simulink model "Phase1_Mark2"  (R2024b)
settings: Solver=ode23tb  StartTime=0.0  StopTime=inf  FixedStep=.001  RelTol=1e-1
model workspace (MAT data in the model file):
  A_mu = 10
  B_reff = 8.386
  CONVERTER_DATA = [0 0.1 0.2 0.3 0.4 0.5 0.6 0.7 0.8 0.81 0.82 0.83 ... (63 elements, 21x3)]
  Cps = 2
  Cz = 7766.25
  DOWN_TABLE = [0 0 0 0 0 0 5 5 7.5 7.5 15 15 ... (30 elements, 6x5)]
  DOWN_TH_BP = [0 5 40 50 90 100]
  D_reff = 0.25826
  EMAP = [-40 215 245 264 264 267 267 267 267 267 -44 117 ... (110 elements, 10x11)]
  F0z = [6086.4 4324.8]
  F_reff = 0.07394
  F_zmax = 10000
  F_zmin = 100
  F_zo = 4000
  Kz = 48000
  MF : object (value not decoded)
  NCyl = 6
  NE_VEC = [800 1200 1600 2000 2400 2800 3200 3600 4000 4400 4800]
  Pstd = 101325
  Rair = 287
  SUS : object (value not decoded)
  TH_VEC = [0; 20; 30; 40; 50; 60; 70; 80; 90; 100]
  TWAITdn = 1.25
  TWAITup = 0.1
  Tin = [1 2 3 4 5 6 7 8 9 10 2 2 ... (20 elements, 10x2)]
  Tstd = 293.15
  UP_TABLE = [7.5 7.5 15 25 40 40 25 25 35 45 70 80 ... (30 elements, 6x5)]
  UP_TH_BP = [0 25 35 50 90 100]
  VEH : object (value not decoded)
  V_o = 16.7
  V_xlow = 1
  Vd = 0.00346
  WH : object (value not decoded)
  a = 1.515
  alpha_max = 1.5
  alpha_min = -1.5
  b = 1.504
  c_zo = 209651
  epsilon = 0.1
  f_air = [0 0 0 0 0 0 0 0 0 0 0 0 ... (256 elements, 16x16)]
  f_co = [0 0 0 0 0 0 0 0 0 0 0 0 ... (256 elements, 16x16)]
  f_co2 = [0 0 0 0 0 0 0 0 0 0 0 0 ... (256 elements, 16x16)]
  f_eff = [352.135682859 352.135682859 320.724378192 303.655312657 295.930136708 291.240087194 291.240271258 291.240312459 291.240275452 291.240198499 291.240100781 291.240018769 ... (256 elements, 16x16)]
  f_fuel = [0 0 0 0 0 0 0 0 0 0 0 0 ... (256 elements, 16x16)]
  f_hc = [0 0 0 0 0 0 0 0 0 0 0 0 ... (256 elements, 16x16)]
  f_nox = [0 0 0 0 0 0 0 0 0 0 0 0 ... (256 elements, 16x16)]
  f_pm = [0 0 0 0 0 0 0 0 0 0 0 0 ... (256 elements, 16x16)]
  f_susp_axl_bp = [1 2]
  f_susp_dz_bp = [-4 -0.14 -0.13 -0.12 -0.11 -0.1 -0.09 -0.08 -0.07 -0.06 -0.05 -0.04 ... (31 elements, 1x31)]
  f_susp_dzdot_bp = [-4 -0.14 -0.13 -0.12 -0.11 -0.1 -0.09 -0.08 -0.07 -0.06 -0.05 -0.04 ... (31 elements, 1x31)]
  f_susp_fmz = [-213379.591456 -28099.591456 -27619.591456 -27139.591456 -26659.591456 -26179.591456 -25699.591456 -25219.591456 -24739.591456 -24259.591456 -23779.591456 -23299.591456 ... (468968 elements, 31x31x61x2x4)]
  f_susp_geom = [-0.832564012244 0.043269987756 0.045538987756 0.047807987756 0.050076987756 0.052345987756 0.054614987756 0.056883987756 0.059152987756 0.061421987756 0.063690987756 0.065959987756 ... (11346 elements, 31x61x2x3)]
  f_susp_strgdelta_bp = [-0.523598775598 -0.506145483078 -0.488692190558 -0.471238898038 -0.453785605519 -0.436332312999 -0.418879020479 -0.401425727959 -0.383972435439 -0.366519142919 -0.349065850399 -0.331612557879 ... (61 elements, 1x61)]
  f_tbrake = [0 76.8593923996 105.140482948 131.533638111 157.926793274 176.658631717 176.65727296 176.656856686 176.656879077 176.657093756 176.657404516 176.65772406 ... (256 elements, 16x16)]
  f_tbrake_n_bpt = [0 649.519052838 912.419621844 1175.32019085 1438.22075986 1701.12132886 1964.02189787 2226.92246687 2489.82303588 2752.72360489 3015.62417389 3278.5247429 ... (16 elements, 1x16)]
  f_tbrake_t_bpt = [0 34.6410161514 61.0341713143 87.4273264773 113.82048164 140.213636803 166.606791966 192.999947129 219.393102292 245.786257455 272.179412618 298.572567781 ... (16 elements, 1x16)]
  f_texh = [766.752464599 766.752464599 786.17542386 801.679939032 884.591982581 910.574397722 910.571871054 910.570774534 910.570601632 910.570821151 910.571247242 910.571639815 ... (256 elements, 16x16)]
  f_twc_eff_co = [0.17 0.25 0.45 0.99 0.99 0.99 0.99]
  f_twc_eff_hc = [0.21 0.375 0.75 0.98 0.98 0.98 0.98]
  f_twc_eff_lam = [0.909090909 0.944055944 0.979020979 1 1.013986014 1.048951049 1.083916084]
  f_twc_eff_nox = [0.98 0.98 0.98 0.97 0.05 0.02 0]
  h = 0.134
  k_z = 50
  kappa_max = 1.5
  kappa_min = -1.5
  lam_Cx = 1
  lam_Cy = 1
  lam_Cz = 1
  lam_Ex = 1
  lam_Ey = 1
  lam_F_zo = 1
  lam_Hx = 1
  lam_Hy = 1
  lam_Kxkappa = 1
  lam_Kyalpha = 1
  lam_Kygamma = 1
  lam_Kzgamma = 1
  lam_Mr = 1
  lam_Mx = 1
  lam_My = 1
  lam_S = 1
  lam_VMx = 1
  lam_Vx = 1
  lam_Vy = 1
  lam_Vykappa = 1
  lam_muV = 0
  lam_mux = 1
  lam_muy = 1
  lam_t = 1
  lam_xalpha = 1
  lam_ykappa = 1
  numWheel = 4
  p_Cx1 = 1.579
  p_Cy1 = 1.3332
  p_Dx1 = 1.0422
  p_Dx2 = -0.08285
  p_Dx3 = 0
  p_Dy1 = 0.8784
  p_Dy2 = -0.06445
  p_Dy3 = 0
  p_Ex1 = 0.11185
  p_Ex2 = 0.3127
  p_Ex3 = 0
  p_Ex4 = 0.001603
  p_Ey1 = -0.8227
  p_Ey2 = -0.6062
  p_Ey3 = 0.09825
  p_Ey4 = -6.546
  p_Ey5 = 0
  p_Fz1 = 0.7098
  p_Hx1 = 0.00021585
  p_Hx2 = 0.0011538
  p_Hy1 = -0.0018043
  p_Hy2 = 0.003518
  p_Kx1 = 21.69
  p_Kx2 = 13.774
  p_Kx3 = -0.4119
  p_Ky1 = -15.314
  p_Ky2 = 1.7044
  p_Ky3 = 0.36986
  p_Ky4 = 1.9896
  p_Ky5 = 0
  p_Ky6 = -0.9004
  p_Ky7 = -0.2328
  p_Vx1 = 1.5973e-05
  p_Vx2 = 0.0001043
  p_Vy1 = -0.006642
  p_Vy2 = 0.03597
  p_Vy3 = -0.1621
  p_Vy4 = -0.4908
  p_pmx1 = 0
  p_px1 = -0.3489
  p_px2 = 0.382
  p_px3 = -0.09634
  p_px4 = 0.06447
  p_py1 = -0.6249
  p_py2 = -0.06535
  p_py3 = -0.1668
  p_py4 = 0.2834
  p_py5 = 0
  path : object (value not decoded)
  pio = 220000
  q_Fcx = 0
  q_Fz2 = 15.4
  q_Fzy = 0
  q_reo = 0.9974
  q_sx1 = -0.007764
  q_sx10 = 0.2824
  q_sx11 = 5.349
  q_sx12 = 0
  q_sx13 = 0
  q_sx14 = 0
  q_sx2 = 1.1915
  q_sx3 = 0.013948
  q_sx4 = 4.912
  q_sx5 = 1.02
  q_sx6 = 22.83
  q_sx7 = 0.7104
  q_sx8 = -0.023393
  q_sx9 = 0.6581
  q_sy1 = 0.00702
  q_sy2 = 0
  q_sy3 = 0.001515
  q_sy4 = 8.514e-05
  q_sy5 = 0
  q_sy6 = 0
  q_sy7 = 0.9008
  q_sy8 = -0.4089
  q_v1 = 0.0007742
  q_v2 = 0.04667
  r_Bx1 = 12.531
  r_Bx2 = 9.532
  r_Bx3 = 0
  r_By1 = 10.615
  r_By2 = 7.705
  r_By3 = 3.433e-06
  r_By4 = 0
  r_Cx1 = 1.019
  r_Cy1 = 1.0585
  r_Ex1 = -0.4487
  r_Ex2 = -0.4726
  r_Ey1 = 0.3132
  r_Ey2 = 7.63e-06
  r_Hx1 = 0.0002374
  r_Hy1 = 0.011646
  r_Hy2 = 7.63e-06
  r_Vy1 = 0.05654
  r_Vy2 = 7.63e-06
  r_Vy3 = 0
  r_Vy4 = 99.9
  r_Vy5 = 2
  r_Vy6 = 15.814
  r_o = 0.3135
  reqTmaxT = [nan 0.285774810084 0.647179872268 nan nan nan nan nan nan nan nan nan ... (168 elements, 21x8)]
  vehSpd = [0 2.77777777778 5.55555555556 8.33333333333 11.1111111111 13.8888888889 16.6666666667 19.4444444444 22.2222222222 25 27.7777777778 30.5555555556 ... (21 elements, 1x21)]
  vehWidth = 2
  w = 1
symbols that are objects in the model workspace (value not decoded): VEH
undefined symbols (not defined in the file or in its folder): Fzz, Fzzdot, InertFrm, pFz, psi, vdyntiremask, x_o, zdotFz, zFz
(part 4 of 24)

== system Phase1_Mark2/Longitudinal Wheels 4DOF/Tires/Fiala ==
  AxlTrq : Inport
  BrkPrs : Inport  Port=2
  Vx : Inport  Port=3
  Vy : Inport  Port=4
  r : Inport  Port=5
  Camber : Inport  Port=6
  TirePrs : Inport  Port=7
  Fz : Inport  Port=8
  Friction : Inport  Port=9
  Ground : Inport  Port=10
  Fiala Tire : Subsystem  InitFcn=%vdyntiremask(gcb,'updateExtAPIButtons');  mask(Fiala Wheel 2DOF){UNLOADED_RADIUS=0.309384029954441, omegao=0, IYY=0.740633832792491, br=1e-3, tireType=User defined, BrakeType=Disc, rollingType=Pressure and velocity, vertType=None, Ckappa=1e4, Calpha=7e4, Cgamma=1e3, muMin=.8, muMax=.9, Lrelx=.01, Lrely=.01, NOMPRES=220000, LONGVL=16, aMy=8e-4, bMy=.001, cMy=1.6e-4, alphaMy=-0.003, betaMy=0.97, QSY1=0.007, QSY2=0, QSY3=0.0015, QSY4=8.5e-05, QSY5=0, QSY6=0, QSY7=0.9, QSY8=-0.4, FNOMIN=4000, lam_My=1, VxMy=-20:1:20, FzMy=0:200:1e4, MyMap=[0,1114.7,4367.1,9707.2,17109,26554,38030,51524,67028,84533,1.0403e+05,1.2552e+05,1.4899e+05,1.7444e+05,2.0185e+05,2.3124e+05,2.6259e+05,2.959e+05,3.3117e+05,3.6839e+05,4.0756e+05,4.4868e+05,4.9174e+05,5.3675e+05,5.8369e+05,6.3257e+05,6.8338e+05,7.3613e+05,7.908e+05,8.474e+05,9.0593e+05,9.6638e+05,1.0288e+06,1.093e+06,1.1593e+06,1.2274e+06,1.2974e+06,1.3694e+06,1.4432e+06,1.519e+06,1.5967e+06,1.6763e+06,1.7578e+06,1.8412e+06,1.9265e+06,2.0137e+06,2.1028e+06,2.1938e+06,2.2867e+06,2.3815e+06,2.4782e+06 0,1024.5,4013.8,8921.9,15725,24406,34953,47356,61605,77694,95616,1.1537e+05,1.3694e+05,1.6032e+05,1.8553e+05,2.1254e+05,2.4135e+05,2.7197e+05,3.0438e+05,3.3859e+05,3.7459e+05,4.1238e+05,4.5196e+05,4.9333e+05,5.3647e+05,5.814e+05,6.281e+05,6.7658e+05,7.2683e+05,7.7885e+05,8.3264e+05,8.8821e+05,9.4553e+05,1.0046e+06,1.0655e+06,1.1281e+06,1.1925e+06,1.2586e+06,1.3265e+06,1.3961e+06,1.4675e+06,1.5407e+06,1.6156e+06,1.6922e+06,1.7706e+06,1.8508e+06,1.9327e+06,2.0163e+06,2.1017e+06,2.1889e+06,2.2777e+06 0,938.57,3677,8173.3,14405,22358,32020,43382,56436,71175,87593,1.0568e+05,1.2545e+05,1.4687e+05,1.6996e+05,1.947e+05,2.211e+05,2.4915e+05,2.7884e+05,3.1018e+05,3.4316e+05,3.7778e+05,4.1404e+05,4.5193e+05,4.9146e+05,5.3261e+05,5.754e+05,6.1981e+05,6.6584e+05,7.135e+05,7.6278e+05,8.1368e+05,8.6619e+05,9.2032e+05,9.7607e+05,1.0334e+06,1.0924e+06,1.153e+06,1.2152e+06,1.279e+06,1.3444e+06,1.4114e+06,1.48e+06,1.5502e+06,1.6221e+06,1.6955e+06,1.7705e+06,1.8471e+06,1.9254e+06,2.0052e+06,2.0866e+06 0,856.81,3356.7,7461.3,13151,20411,29231,39603,51520,64974,79962,96478,1.1452e+05,1.3408e+05,1.5515e+05,1.7774e+05,2.0184e+05,2.2744e+05,2.5455e+05,2.8316e+05,3.1327e+05,3.4487e+05,3.7797e+05,4.1256e+05,4.4864e+05,4.8621e+05,5.2527e+05,5.6581e+05,6.0784e+05,6.5134e+05,6.9633e+05,7.4279e+05,7.9073e+05,8.4015e+05,8.9104e+05,9.4341e+05,9.9724e+05,1.0525e+06,1.1093e+06,1.1676e+06,1.2273e+06,1.2885e+06,1.3511e+06,1.4152e+06,1.4808e+06,1.5478e+06,1.6163e+06,1.6862e+06,1.7576e+06,1.8305e+06,1.9048e+06 0,779.25,3052.9,6785.9,11960,18563,26585,36018,46856,59093,72724,87745,1.0415e+05,1.2194e+05,1.4111e+05,1.6165e+05,1.8357e+05,2.0685e+05,2.3151e+05,2.5753e+05,2.8491e+05,3.1365e+05,3.4376e+05,3.7522e+05,4.0803e+05,4.422e+05,4.7772e+05,5.1459e+05,5.5282e+05,5.9238e+05,6.333e+05,6.7556e+05,7.1916e+05,7.641e+05,8.1039e+05,8.5801e+05,9.0697e+05,9.5727e+05,1.0089e+06,1.0619e+06,1.1162e+06,1.1718e+06,1.2288e+06,1.2871e+06,1.3467e+06,1.4077e+06,1.47e+06,1.5336e+06,1.5985e+06,1.6648e+06,1.7324e+06 0,705.9,2765.5,6147.1,10834,16816,24083,32628,42446,53531,65879,79486,94348,1.1046e+05,1.2783e+05,1.4643e+05,1.6629e+05,1.8738e+05,2.0972e+05,2.3329e+05,2.5809e+05,2.8413e+05,3.114e+05,3.399e+05,3.6962e+05,4.0058e+05,4.3276e+05,4.6616e+05,5.0078e+05,5.3662e+05,5.7369e+05,6.1197e+05,6.5146e+05,6.9218e+05,7.3411e+05,7.7725e+05,8.216e+05,8.6717e+05,9.1394e+05,9.6193e+05,1.0111e+06,1.0615e+06,1.1131e+06,1.1659e+06,1.22e+06,1.2752e+06,1.3316e+06,1.3892e+06,1.4481e+06,1.5081e+06,1.5693e+06 0,636.76,2494.6,5545,9773.1,15169,21724,29432,38288,48287,59426,71700,85106,99642,1.153e+05,1.3209e+05,1.5e+05,1.6903e+05,1.8917e+05,2.1044e+05,2.3281e+05,2.563e+05,2.809e+05,3.066e+05,3.3342e+05,3.6134e+05,3.9037e+05,4.205e+05,4.5173e+05,4.8406e+05,5.1749e+05,5.5202e+05,5.8765e+05,6.2438e+05,6.622e+05,7.0111e+05,7.4112e+05,7.8223e+05,8.2442e+05,8.677e+05,9.1208e+05,9.5754e+05,1.0041e+06,1.0517e+06,1.1005e+06,1.1503e+06,1.2012e+06,1.2532e+06,1.3062e+06,1.3604e+06,1.4156e+06 0,571.82,2240.2,4979.5,8776.4,13622,19508,26430,34383,43363,53365,64388,76427,89480,1.0355e+05,1.1862e+05,1.347e+05,1.5179e+05,1.6988e+05,1.8897e+05,2.0907e+05,2.3016e+05,2.5225e+05,2.7534e+05,2.9942e+05,3.2449e+05,3.5056e+05,3.7761e+05,4.0566e+05,4.3469e+05,4.6472e+05,4.9573e+05,5.2772e+05,5.607e+05,5.9467e+05,6.2961e+05,6.6554e+05,7.0245e+05,7.4034e+05,7.7921e+05,8.1906e+05,8.5989e+05,9.017e+05,9.4448e+05,9.8824e+05,1.033e+06,1.0787e+06,1.1254e+06,1.173e+06,1.2216e+06,1.2712e+06 0,511.09,2002.3,4450.7,7844.3,12175,17436 ...(+15095 chars)], Fpl=10, Cr=1e-3, Kt=.008, Tmeas=298.15, Tamb=298.15, extTamb=off, WIDTH=0.209045013245853, bMz=0, mu_static=.3, mu_kinetic=.2, disk_abore=.05, Rm=.177, num_pads=2, drum_abore=0.0508, drum_a=0.123, drum_c=0.212, drum_r=0.15, drum_theta1=0, drum_theta2=126, brake_p_bpt=[1 11.4736842105263 21.9473684210526 32.4210526315789 42.8947368421053 53.3684210526316 63.8421052631579 74.3157894736842 84.7894736842105 95.2631578947368 105.736842105263 116.210526315789 126.684210526316 137.157894736842 147.631578947368 158.105263157895 168.578947368421 179.052631578947 189.526315789474 200], brake_n_bpt=[0 52.6315789473684 105.263157894737 157.894736842105 210.526315789474 263.157894736842 315.789473684211 368.421052631579 421.052631578947 473.684210526316 526.315789473684 578.947368421053 631.578947368421 684.210526315789 736.842105263158 789.473684210526 842.105263157895 894.736842105263 947.368421052632 1000], f_brake_t=[43.4900602404453 42.5056030554862 41.5350898940194 40.5780454442085 39.6340111501808 38.7025443887544 37.7832176914519 36.8756180088306 35.9793460143796 35.0940154454303 34.2192524787115 33.3546951383474 32.4999927342521 31.6548053290159 30.8188032315107 29.991666515561 29.1730845621415 28.362755623661 27.5603864089927 26.765691687993;498.991217495636 487.695866636631 476.560505099801 465.579679307235 454.748127933653 444.060772460445 433.51270824929 423.099196101319 412.81565427025 402.657650900201 392.620896861006 382.701238955775 372.894653477208 363.197240090814 353.605216024701 344.114910546964 334.722759712992 325.425301366216 316.219170376863 307.10109410434;954.492374750826 932.886130217776 911.585920305583 890.581313170261 869.862244717126 849.419000532136 829.242198807128 809.322774193808 789.651962526121 770.221286354971 751.0225412433 732.047782773203 713.289314220164 694.739674852612 676.391628817892 658.238154578366 640.272434863842 622.48784710877 604.877954344734 587.436496520688;1409.99353200602 1378.07639379892 1346.61133551136 1315.58294703329 1284.9763615006 1254.77722860383 1224.97168936497 1195.5463522863 1166.48827078199 1137.78492180974 1109.42418562559 1081.39432659063 1053.68397496312 1026.28210961441 999.178041611083 972.361398609768 945.822110014692 919.550392851325 893.536738312604 867.771898937035;1865.49468926121 1823.26665738007 1781.63675071715 1740.58458089631 1700.09047828407 1660.13545667552 1620.7011799228 1581.76993037878 1543.32457903786 1505.34855726451 1467.82583000789 1430.74087040806 1394.07863570608 1357.82454437621 1321.96445440427 1286.48464264117 1251.37178516554 1216.61293859388 1182.19552228048 1148.10730135338;2320.9958465164 2268.45692096121 2216.66216592293 2165.58621475934 2115.20459506754 2065.49368474721 2016.43067048064 1967.99350847127 1920.16088729373 1872.91219271928 1826.22747439018 1780.08741422549 1734.47329644903 1689.36697913801 1644.75086719747 1600.60788667257 1556.92146031639 1513.67548433643 1470.85430624835 1428.44270376973;2776.49700377159 2713.64718454235 2651.68758112871 2590.58784862237 2530.31871185102 2470.8519128189 2412.16016103848 2354.21708656376 2296.9971955496 2240.47582817405 2184.62911877248 2129.43395804292 2074.86795719199 2020.9094138998 1967.53727999066 1914.73113070398 1862.47113546724 1810.73803007899 1759.51309021622 1708.77810618608;3231.99816102678 3158.8374481235 3086.71299633449 3015.58948248539 2945.43282863449 2876.21014089059 2807.88965159632 2740.44066465625 2673.83350380547 2608.03946362882 2543.03076315477 2478.78050186034 2415.26261793494 2352.4518486616 2290.32369278385 2228.85437473538 2168.02081061809 2107.80057582154 2048.17187418409 1989.11350860242;3687.49931828197 3604.02771170464 3521.73841154027 3440.59111634842 3360.54694541796 3281.56836896228 3203.61914215416 3126.66424274874 3050.66981206134 2975.60309908359 2901.43240753707 2828.12704567777 2755.6572786779 2683.9942834234 2613.11010557704 2542.97761876678 2473.57048576894 2404.8631215641 2336.83065815196 2269.44891101877;4143.00047553716 4049.21797528579 3956.76382674606 3865.59275021144 3775.66106220143 3686.92659703397 3599.34863271199 3512.88782084123 3427.50612031721 3343.16673453836 3259.83405191936 3177.4735894952 3096.05193942085 3015.5367181852 2935.89651837023 2857.10086279818 2779.12016091979 2701.92566730665 2625.48944211983 2549.78431343512;4598.50163279235 4494.40823886693 4391.78924195184 4290.59438407447 4190.77517898491 4092.28482510566 3995.07812326983 3899.11139893372 3804.34242857308 3710.73036999313 3618.23569630166 3526.82013331263 3436.44660016381 3347.079152947 3258.68293116342 3171.22410682959 3084.66983607064 2998.98821304921 2914.1482260877 2830.11971585147;5054.00279004754 4939.59850244808 4826.81465715762 4715.59601793749 4605.88929576838 4497.64305317735 4390.80761382767 4285.3349770262 4181.17873682896 4078.2940054479 3976.63734068395 3876.16667713006 3776.84126090677 3678.62158770879 3581.46934395661 3485.34735086099 ...(+2764 chars)], MASS=9.46491996974568, zo=0, zdoto=0, GRAVITY=-9.81, VERTICAL_DAMPING=500, VERTICAL_STIFFNESS=207885, zFz=[0 .01 .1], pFz=[10000 1000000], Fzz=[0 1e3 1e4; 0 1e4 1e5], zdotFz=[-20 0 20], Fzzdot=[500 0 -500;250 0 -250], FZMAX=10000, FZMIN=100, PRESMAX=1003118.65547859, PRESMIN=9982.11955979412, KPUMAX=1.48764378595932, KPUMIN=-1.48007456759542, ALPMAX=1.47424202250808, ALPMIN=-1.50806269049027, CAMMAX=0.173142086627737, CAMMIN=-0.173348165334087, TMIN=0, TMAX=400, aMode=2, MyRelFreqLwrLim=100*pi}
      mask prompts: UNLOADED_RADIUS "vdynblks:vehdynLatTire:blkPrm_UNLOADED_RADIUS"; omegao "vdynblks:vehdynLatTire:blkPrm_omegao"; IYY "vdynblks:vehdynLatTire:blkPrm_IYY"; br "vdynblks:vehdynLatTire:blkPrm_br"; tireType "vdynblks:vehdynLatTire:blkPrm_tireType"; BrakeType "vdynblks:vehdynLatTire:blkPrm_BrakeType"; rollingType "autoblks_shared:autoblkLongitudinalWheel:blkPrm_rollingType"; vertType "vdynblks:vehdyntireFiala:blkPrm_vertType"; Ckappa "vdynblks:vehdyntireFiala:blkPrm_Ckappa"; Calpha "vdynblks:vehdyntireFiala:blkPrm_Calpha"; Cgamma "vdynblks:vehdyntireFiala:blkPrm_Cgamma"; muMin "vdynblks:vehdyntireFiala:blkPrm_muMin"; muMax "vdynblks:vehdyntireFiala:blkPrm_muMax"; Lrelx "vdynblks:vehdyntireFiala:blkPrm_Lrelx"; Lrely "vdynblks:vehdyntireFiala:blkPrm_Lrely"; NOMPRES "autoblks_shared:autoblkLongitudinalWheel:blkPrm_NOMPRES"; LONGVL "autoblks_shared:autoblkLongitudinalWheel:blkPrm_LONGVL"; aMy "vdynblks:vehdyntireFiala:blkPrm_aMy"; bMy "vdynblks:vehdyntireFiala:blkPrm_bMy"; cMy "vdynblks:vehdyntireFiala:blkPrm_cMy"; alphaMy "vdynblks:vehdyntireFiala:blkPrm_alphaMy"; betaMy "vdynblks:vehdyntireFiala:blkPrm_betaMy"; QSY1 "autoblks_shared:autoblkLongitudinalWheel:blkPrm_QSY1"; QSY2 "autoblks_shared:autoblkLongitudinalWheel:blkPrm_QSY2"; QSY3 "autoblks_shared:autoblkLongitudinalWheel:blkPrm_QSY3"; QSY4 "autoblks_shared:autoblkLongitudinalWheel:blkPrm_QSY4"; QSY5 "autoblks_shared:autoblkLongitudinalWheel:blkPrm_QSY5"; QSY6 "autoblks_shared:autoblkLongitudinalWheel:blkPrm_QSY6"; QSY7 "autoblks_shared:autoblkLongitudinalWheel:blkPrm_QSY7"; QSY8 "autoblks_shared:autoblkLongitudinalWheel:blkPrm_QSY8"; FNOMIN "autoblks_shared:autoblkLongitudinalWheel:blkPrm_FNOMIN"; lam_My "autoblks_shared:autoblkLongitudinalWheel:blkPrm_lam_My"; VxMy "autoblks_shared:autoblkLongitudinalWheel:blkPrm_VxMy"; FzMy "autoblks_shared:autoblkLongitudinalWheel:blkPrm_FzMy"; MyMap "autoblks_shared:autoblkLongitudinalWheel:blkPrm_MyMap"; Fpl "autoblks_shared:autoblkLongitudinalWheel:blkPrm_Fpl"; Cr "autoblks_shared:autoblkLongitudinalWheel:blkPrm_Cr"; Kt "autoblks_shared:autoblkLongitudinalWheel:blkPrm_Kt"; Tmeas "autoblks_shared:autoblkLongitudinalWheel:blkPrm_Tmeas"; Tamb "autoblks_shared:autoblkLongitudinalWheel:blkPrm_Tamb"; extTamb "autoblks_shared:autoblkLongitudinalWheel:blkPrm_extTamb"; WIDTH "vdynblks:vehdynLatTire:blkPrm_WIDTH"; bMz "vdynblks:vehdyntireFiala:blkPrm_bMz"; mu_static "autoblks_shared:autoblkLongitudinalWheel:blkPrm_mu_static"; mu_kinetic "autoblks_shared:autoblkLongitudinalWheel:blkPrm_mu_kinetic"; disk_abore "autoblks_shared:autoblkLongitudinalWheel:blkPrm_disk_abore"; Rm "autoblks_shared:autoblkLongitudinalWheel:blkPrm_Rm"; num_pads "autoblks_shared:autoblkLongitudinalWheel:blkPrm_num_pads"; drum_abore "autoblks_shared:autoblkLongitudinalWheel:blkPrm_drum_abore"; drum_a "autoblks_shared:autoblkLongitudinalWheel:blkPrm_drum_a"; drum_c "autoblks_shared:autoblkLongitudinalWheel:blkPrm_drum_c"; drum_r "autoblks_shared:autoblkLongitudinalWheel:blkPrm_drum_r"; drum_theta1 "autoblks_shared:autoblkLongitudinalWheel:blkPrm_drum_theta1"; drum_theta2 "autoblks_shared:autoblkLongitudinalWheel:blkPrm_drum_theta2"; brake_p_bpt "autoblks_shared:autoblkLongitudinalWheel:blkPrm_brake_p_bpt"; brake_n_bpt "autoblks_shared:autoblkLongitudinalWheel:blkPrm_brake_n_bpt"; f_brake_t "autoblks_shared:autoblkLongitudinalWheel:blkPrm_f_brake_t"; MASS "vdynblks:vehdynLatTire:blkPrm_MASS"; zo "vdynblks:vehdynLatTire:blkPrm_zo"; zdoto "vdynblks:vehdynLatTire:blkPrm_zdoto"; GRAVITY "vdynblks:vehdynLatTire:blkPrm_GRAVITY"; VERTICAL_DAMPING "vdynblks:vehdynLatTire:blkPrm_VERTICAL_DAMPING"; VERTICAL_STIFFNESS "vdynblks:vehdynLatTire:blkPrm_VERTICAL_STIFFNESS"; zFz "vdynblks:vehdyntireFiala:blkPrm_zFz"; pFz "vdynblks:vehdyntireFiala:blkPrm_pFz"; Fzz "vdynblks:vehdyntireFiala:blkPrm_Fzz"; zdotFz "vdynblks:vehdyntireFiala:blkPrm_zdotFz"; Fzzdot "vdynblks:vehdyntireFiala:blkPrm_Fzzdot"; FZMAX "vdynblks:vehdynLatTire:blkPrm_FZMAX"; FZMIN "vdynblks:vehdynLatTire:blkPrm_FZMIN"; PRESMAX "vdynblks:vehdynLatTire:blkPrm_PRESMAX"; PRESMIN "vdynblks:vehdynLatTire:blkPrm_PRESMIN"; KPUMAX "vdynblks:vehdynLatTire:blkPrm_KPUMAX"; KPUMIN "vdynblks:vehdynLatTire:blkPrm_KPUMIN"; ALPMAX "vdynblks:vehdynLatTire:blkPrm_ALPMAX"; ALPMIN "vdynblks:vehdynLatTire:blkPrm_ALPMIN"; CAMMAX "vdynblks:vehdynLatTire:blkPrm_CAMMAX"; CAMMIN "vdynblks:vehdynLatTire:blkPrm_CAMMIN"; TMIN "autoblks_shared:autoblkLongitudinalWheel:blkPrm_TMIN"; TMAX "autoblks_shared:autoblkLongitudinalWheel:blkPrm_TMAX"; MyRelFreqLwrLim "Rolling relaxation length lower frequency limit, MyRelFreqLwrLim [rad/s]:"
      mask help: vdynblks:vehdyntireFiala:blkDesc
      mask init:
      | [~]=vehdynicon('vehdynlibtirefiala',gcb,0);
      mask Help: eval('vdynblkshelp(''vbtirefiala'')')
      mask Callback tireType: [~]=vehdynicon('vehdynlibtirefiala',gcb,6);
      mask TypeOptions BrakeType: autoblks_shared:autoblkLongitudinalWheel:blkCmb_BrakeType_c1 | autoblks_shared:autoblkLongitudinalWheel:blkCmb_BrakeType_c2 | autoblks_shared:autoblkLongitudinalWheel:blkCmb_BrakeType_c3 | autoblks_shared:autoblkLongitudinalWheel:blkCmb_BrakeType_c4
      mask Callback BrakeType: [~]=vehdynicon('vehdynlibtirefiala',gcb,2);
      mask TypeOptions rollingType: autoblks_shared:autoblkLongitudinalWheel:blkCmb_rollingType_c1 | autoblks_shared:autoblkLongitudinalWheel:blkCmb_rollingType_c2 | autoblks_shared:autoblkLongitudinalWheel:blkCmb_rollingType_c5 | autoblks_shared:autoblkLongitudinalWheel:blkCmb_rollingType_c3 | autoblks_shared:autoblkLongitudinalWheel:blkCmb_rollingType_c4
      mask Callback rollingType: [~]=vehdynicon('vehdynlibtirefiala',gcb,1);
      mask TypeOptions vertType: vdynblks:vehdyntireFiala:blkCmb_vertType_c1 | vdynblks:vehdyntireFiala:blkCmb_vertType_c2 | vdynblks:vehdyntireFiala:blkCmb_vertType_c3
      mask Callback vertType: [~]=vehdynicon('vehdynlibtirefiala',gcb,5);
      mask DialogControl BlockOptions Prompt: autoblks_shared:autoblkLongitudinalWheel:blkDlg_BlockOptions
      mask DialogControl SourceOptions Prompt: vdynblks:vehdynLatTire:blkDlg_SourceOptions
      mask DialogControl tireType Prompt: Tire type:
      mask DialogControl paramOverwrite Prompt: vdynblks:vehdynLatTire:blkPrm_paramOverwrite
      mask DialogControl paramOverwrite Callback: [~]=vehdynicon('vehdynlibtirefiala',gcb,7);
      mask DialogControl BrakeType Prompt: Brake type:
      mask DialogControl rollingType Prompt: Rolling Resistance:
      mask DialogControl vertType Prompt: Vertical Motion:
      mask DialogControl WheelParams Prompt: vdynblks:vehdynLatTire:blkDlg_WheelParams
      mask DialogControl longlatParamPanel Prompt: vdynblks:vehdyntireFiala:blkPrm_longlatParamPanel
      mask DialogControl Ckappa Prompt: Longitudinal stiffness, Ckappa [N]:
      mask DialogControl Calpha Prompt: Lateral stiffness per slip angle, Calpha [N/rad]:
      mask DialogControl Cgamma Prompt: Camber stiffness, Cgamma [N/rad]:
      mask DialogControl muMin Prompt: Kinematic friction, muMin []:
      mask DialogControl muMax Prompt: Static friction, muMax []:
      mask DialogControl Lrelx Prompt: Longitudinal relaxation length, Lrelx [m]:
      mask DialogControl Lrely Prompt: Lateral relaxation length, Lrely [m/rad]:
      mask DialogControl rollingParamPanel Prompt: autoblks_shared:autoblkLongitudinalWheel:blkDlg_rollingParamPanel
      mask DialogControl NOMPRES Prompt: Nominal inflation pressure, NOMPRES [Pa]:
      mask DialogControl LONGVL Prompt: Nominal longitudinal speed, LONGVL [m/s]:
      mask DialogControl SimpMyParams Prompt: autoblks_shared:autoblkLongitudinalWheel:blkDlg_SimpMyParams
      mask DialogControl aMy Prompt: Velocity independent force coefficient, aMy []:
      mask DialogControl bMy Prompt: Linear velocity force component, bMy [s/m]:
      mask DialogControl cMy Prompt: Quadratic velocity force component, cMy [s^2/m^2]:
      mask DialogControl alphaMy Prompt: Tire pressure exponent, alphaMy []:
      mask DialogControl betaMy Prompt: Normal force exponent, betaMy []:
      mask DialogControl MagicMyParams Prompt: autoblks_shared:autoblkLongitudinalWheel:blkDlg_MagicMyParams
      mask DialogControl QSY1 Prompt: Rolling resistance torque coefficient, QSY1 []:
      mask DialogControl QSY2 Prompt: Longitudinal force rolling resistance coefficient, QSY2 []:
      mask DialogControl QSY3 Prompt: Linear rotational speed rolling resistance coefficient, QSY3 []:
      mask DialogControl QSY4 Prompt: Quartic rotational speed rolling resistance coefficient, QSY4 []:
      mask DialogControl QSY5 Prompt: Camber squared rolling resistance torque, QSY5 [1/rad^2]:
      mask DialogControl QSY6 Prompt: Load based camber squared rolling resistance torque, QSY6 [1/rad^2]:
      mask DialogControl QSY7 Prompt: Normal load rolling resistance coefficient, QSY7 []:
      mask DialogControl QSY8 Prompt: Pressure load rolling resistance coefficient, QSY8 []:
      mask DialogControl FNOMIN Prompt: Nominal normal force, FNOMIN [N]:
      mask DialogControl lam_My Prompt: Rolling resistance scaling factor, lam_My []:
      mask DialogControl MappedMyParams Prompt: autoblks_shared:autoblkLongitudinalWheel:blkDlg_MappedMyParams
      mask DialogControl VxMy Prompt: Spin axis velocity breakpoints, VxMy [m/s]:
      mask DialogControl FzMy Prompt: Normal force breakpoints, FzMy [N]:
      mask DialogControl MyMap Prompt: Rolling resistance torque map, MyMap [Nm]:
      mask DialogControl plotMyMap Prompt: autoblks_shared:autoblkLongitudinalWheel:blkDlg_plotMyMap
      mask DialogControl plotMyMap Callback: [~]=vehdynicon('vehdynlibtirefiala',gcb,4);
      mask DialogControl ISOMyParams Prompt: autoblks_shared:autoblkLongitudinalWheel:blkDlg_ISOMyParams
      mask DialogControl Fpl Prompt: Parasitic losses force, Fpl [N]:
      mask DialogControl Cr Prompt: Rolling resistance constant, Cr [N/kN]:
      mask DialogControl Kt Prompt: Thermal correction factor, Kt [1/degC]:
      mask DialogControl Tmeas Prompt: Measured temperature, Tmeas [K]:
      mask DialogControl Tamb Prompt: Ambient temperature, Tamb [K]:
      mask DialogControl extTamb Prompt: Input ambient temperature
      mask DialogControl alignParamPannel Prompt: vdynblks:vehdynLatTire:blkDlg_alignParamPanel
      mask DialogControl WIDTH Prompt: Tire nominal section width, WIDTH [m]:
      mask DialogControl bMz Prompt: Linear yaw rate resistance, bMz [N*m*s/rad]:
      mask DialogControl brakeParamPanel Prompt: autoblks_shared:autoblkLongitudinalWheel:blkDlg_brakeParamPanel
      mask DialogControl GenParams Prompt: autoblks_shared:autoblkLongitudinalWheel:blkDlg_GenParams
      mask DialogControl mu_static Prompt: Static friction coefficient, mu_static []:
      mask DialogControl mu_kinetic Prompt: Kinetic friction coefficient, mu_kinetic []:
      mask DialogControl DiskBrakeParms Prompt: autoblks_shared:autoblkLongitudinalWheel:blkDlg_DiskBrakeParms
      mask DialogControl disk_abore Prompt: Disc brake actuator bore, disk_abore [m]:
      mask DialogControl Rm Prompt: Brake pad mean radius, Rm [m]:
      mask DialogControl num_pads Prompt: Number of brake pads, num_pads []:
      mask DialogControl DrumBrakeParms Prompt: autoblks_shared:autoblkLongitudinalWheel:blkDlg_DrumBrakeParms
      mask DialogControl drum_abore Prompt: Drum brake actuator bore, drum_abore [m]:
      mask DialogControl drum_a Prompt: Shoe pin to drum center distance, drum_a [m]:
      mask DialogControl drum_c Prompt: Shoe pin center to force application point distance, drum_c [m]:
      mask DialogControl drum_r Prompt: Drum internal radius, drum_r [m]:
      mask DialogControl drum_theta1 Prompt: Shoe pin to pad start angle, drum_theta1 [deg]:
      mask DialogControl drum_theta2 Prompt: Shoe pin to pad end angle, drum_theta2 [deg]:
      mask DialogControl MappedBrakeParms Prompt: autoblks_shared:autoblkLongitudinalWheel:blkDlg_MappedBrakeParms
      mask DialogControl brake_p_bpt Prompt: Brake actuator pressure breakpoints, brake_p_bpt [bar]:
      mask DialogControl brake_n_bpt Prompt: Wheel speed breakpoints, brake_n_bpt [rpm]:
      mask DialogControl f_brake_t Prompt: Brake torque map, f_brake_t [Nm]:
      mask DialogControl PlotBrakeTorqueMap Prompt: autoblks_shared:autoblkLongitudinalWheel:blkDlg_PlotBrakeTorqueMap
      mask DialogControl PlotBrakeTorqueMap Callback: [~]=vehdynicon('vehdynlibtirefiala',gcb,3);
      mask DialogControl vertParamPannel Prompt: autoblks_shared:autoblkLongitudinalWheel:blkDlg_vertDynParamPanel
      mask DialogControl MASS Prompt: Tire mass, MASS [kg]:
      mask DialogControl zo Prompt: Initial tire displacement, zo [m]:
      mask DialogControl zdoto Prompt: Initial wheel vertical velocity (wheel fixed frame), zdoto [m/s]:
      mask DialogControl GRAVITY Prompt: Gravity, GRAVITY [m/s^2]:
      mask DialogControl vertLinearParam Prompt: vdynblks:vehdyntireFiala:blkDlg_vertLinearParam
      mask DialogControl VERTICAL_DAMPING Prompt: Vertical tire damping, VERTICAL_DAMPING [N*s/m]:
      mask DialogControl VERTICAL_STIFFNESS Prompt: Vertical tire stiffness, VERTICAL_STIFFNESS [N/m]:
      mask DialogControl vertMappedParam Prompt: autoblks_shared:autoblkLongitudinalWheel:blkDlg_vertMappedParam
      mask DialogControl zFz Prompt: Vertical deflection breakpoints, zFz [m]:
      mask DialogControl pFz Prompt: Pressure breakpoints, pFz [Pa]:
      mask DialogControl Fzz Prompt: Force due to deflection, Fzz [N]:
      mask DialogControl zdotFz Prompt: Vertical velocity breakpoints, zdotFz [m/s]:
      mask DialogControl Fzzdot Prompt: Force due to velocity, Fzzdot [N]:
      mask DialogControl WheelParam Prompt: vdynblks:vehdyntireFiala:blkDlg_WheelParams
      mask DialogControl UNLOADED_RADIUS Prompt: Tire unloaded radius, UNLOADED_RADIUS [m]:
      mask DialogControl omegao Prompt: Initial wheel rotational velocity, omegao [rad/s]:
      mask DialogControl IYY Prompt: Tire rotational inertia (rolling axis), IYY [kg*m^2]:
      mask DialogControl br Prompt: Rotational damping, br [N*m*s/rad]:
      mask DialogControl simParamPannel Prompt: autoblks_shared:autoblkLongitudinalWheel:blkDlg_simParamPanel
      mask DialogControl FZMAX Prompt: Maximum normal force, FZMAX [N]:
      mask DialogControl FZMIN Prompt: Minimum normal force, FZMIN [N]:
      mask DialogControl PRESMAX Prompt: Maximum pressure, PRESMAX [Pa]:
      mask DialogControl PRESMIN Prompt: Minimum pressure, PRESMIN [Pa]:
      mask DialogControl KPUMAX Prompt: Max allowable slip ratio (absolute), KPUMAX []:
      mask DialogControl KPUMIN Prompt: Minimum allowable slip ratio (absolute), KPUMIN []:
      mask DialogControl ALPMAX Prompt: Max allowable slip angle (absolute), ALPMAX [rad]:
      mask DialogControl ALPMIN Prompt: Minimum allowable slip angle (absolute), ALPMIN [rad]:
      mask DialogControl CAMMAX Prompt: Maximum allowable camber angle, CAMMAX [rad]:
      mask DialogControl CAMMIN Prompt: Minimum allowable camber angle, CAMMIN [rad]:
      mask DialogControl TMIN Prompt: Minimum ambient temperature, TMIN, [K]:
      mask DialogControl TMAX Prompt: Maximum ambient temperature, TMAX [K]:
      mask DialogControl plotGroup Prompt: vdynblks:vehdynLatTire:blkDlg_Plotting
      mask DialogControl plotTireFM Prompt: vdynblks:vehdynLatTire:blkPrm_plotTireFM
      mask DialogControl plotTireFM Callback: [~]=vehdynicon('vehdynlibtirefiala',gcb,11);
      mask DialogControl getTireAPIs Prompt: vdynblks:vehdynLatTire:blkPrm_getTireAPIs
      mask DialogControl getTireAPIs Callback: [~]=vehdynicon('vehdynlibtirefiala',gcb,10);
      mask Display:
      | try
      |     IconInfo = vehdynicon('vehdynlibtirefiala',gcb,8);
      | 
      |     image(IconInfo.image, IconInfo.position);
      | 
      |     for i = 1:numel(IconInfo.lconn)
      |         port_label('lconn', i, IconInfo.lconn{i})
      |     end
      | 
      |     for j = 1:numel(IconInfo.rconn)
      |         port_label('rconn', j, IconInfo.rconn{j})
      |     end
      | 
      |     for k = 1:numel(IconInfo.input)
      |         port_label('input', k, IconInfo.input{k})
      |     end
      | 
      |     for m = 1:numel(IconInfo.output)
      |         port_label('output', m, IconInfo.output{m})
      |     end
      | catch
      |     fprintf('2DOF \n Wheel')
      | end
  Terminator{,1..6} (7 alike) : Terminator
  Wheel : Outport  VectorParamsAs1DForOutWhenUnconnected=off
  wires:
  Fiala Tire/1(Info) -> Wheel/1
  Camber/1 -> Fiala Tire/5(Camber)
  r/1 -> Fiala Tire/6(YawRate)
  Vy/1 -> Fiala Tire/4(Vy)
  AxlTrq/1 -> Fiala Tire/2(AxlTrq)
  BrkPrs/1 -> Fiala Tire/1(BrkPrs)
  Vx/1 -> Fiala Tire/3(Vx)
  TirePrs/1 -> Fiala Tire/7(Prs)
  Ground/1 -> Fiala Tire/8(Gnd)
  Fz/1 -> Fiala Tire/9(Fext)
  Friction/1 -> Fiala Tire/10(ScaleFctr)
  Fiala Tire/2(Omega) -> Terminator/1
  Fiala Tire/3(Fx) -> Terminator1/1
  Fiala Tire/5(Fz) -> Terminator3/1
  Fiala Tire/4(Fy) -> Terminator2/1
  Fiala Tire/8(Mz) -> Terminator6/1
  Fiala Tire/7(My) -> Terminator5/1
  Fiala Tire/6(Mx) -> Terminator4/1
